simulink model "torque_controller_subsystem_completed_V2_R2019"  (R2019a)
settings: Solver=VariableStepAuto  StartTime=0.0  StopTime=5  RelTol=1e-3
model workspace (MAT data in the model file):
  DCBusVoltage = 24
  K_e = 221.0633
  L_d = 0.003482
  L_q = 0.00456
  Machine_Temperature = 25
  N = 9
  Peak_Current_String = 'Peak Current = 6.000000'
  PhaseAdvancesPerCycle = 36
  Phase_Advance_String = 'PhaseAdvance = 180.000000'
  PointsPerCycle = 36
  Rload = 1000000
  Rs = 0.624570538244
  Shaft_Speed = 27
  Sig = Simulink.Signal
  Sig.DataType = 'auto'
  Sig.Dimensions = -1
  Sig.DimensionsMode = 'auto'
  Sig.Complexity = 'auto'
  Sig.SampleTime = -1
  Sig.SamplingMode = 'auto'
  Sig1 = Simulink.Signal
  Sig1.DataType = 'auto'
  Sig1.Dimensions = -1
  Sig1.DimensionsMode = 'auto'
  Sig1.Complexity = 'auto'
  Sig1.SampleTime = -1
  Sig1.SamplingMode = 'auto'
  angleVec = [0 1.11111111111 2.22222222222 3.33333333333 4.44444444444 5.55555555556 6.66666666667 7.77777777778 8.88888888889 10 11.1111111111 12.2222222222 13.3333333333 14.4444444444 15.5555555556 16.6666666667 17.7777777778 18.8888888889 20 21.1111111111 22.2222222222 23.3333333333 24.4444444444 25.5555555556 26.6666666667 27.7777777778 28.8888888889 30 31.1111111111 32.2222222222 33.3333333333 34.4444444444 35.5555555556 36.6666666667 37.7777777778 38.8888888889 40]
  dq_inductance = 0.008366
  fluxAmat = [5.78758604472e-05 -0.00245230641441 -0.00496086974489 -0.00746825845512 -0.00997085180846 -0.0124701917234 -0.0149650380151 -0.0174527751443 -0.0199339133996 -0.0224017046643 -0.0248570910938 -0.0273006981398 ... (16428 elements, 12x37x37)]
  fluxD = 0.129208614948
  fluxDmat = [0.129332720835 0.129331856309 0.129330386347 0.129326055027 0.129320008491 0.129311398581 0.12929964601 0.129284600324 0.129267743431 0.129250546721 0.129230887735 0.129208614948 ... (16428 elements, 12x37x37)]
  fluxQ = -0.0273006981398
  fluxQmat = [5.78758604472e-05 -0.00245230641441 -0.00496086974489 -0.00746825845512 -0.00997085180846 -0.0124701917234 -0.0149650380151 -0.0174527751443 -0.0199339133996 -0.0224017046643 -0.0248570910938 -0.0273006981398 ... (16428 elements, 12x37x37)]
  fluxes = [-0.0273006981398; -0.0982475938625; 0.125548292002]
  funcresult = 0
  gammaVec = [-180 -170 -160 -150 -140 -130 -120 -110 -100 -90 -80 -70 -60 -50 -40 -30 -20 -10 0 10 20 30 40 50 60 70 80 90 100 110 120 130 140 150 160 170 180]
  i = 12
  invP = [-2.44929359829e-16  1; -0.866025403784  -0.5; 0.866025403784  -0.5]
  j = 37
  m = 37
  magVec = [0 0.545454545455 1.09090909091 1.63636363636 2.18181818182 2.72727272727 3.27272727273 3.81818181818 4.36363636364 4.90909090909 5.45454545455 6]
  nGamma = 37
  nMag = 12
  nX = 37
  poleNumber = 18
  pole_pairs = 9
  res1 = 0
  res2 = 0
  res3 = 0
  resistance_per_phase = 0.6246
  torque = -10.6713070894
  torqueMat = [-0.000127780443833 -0.972425785337 -1.94471415001 -2.91686171491 -3.8887574387 -4.86000619896 -5.83073162472 -6.80075888771 -7.77012767412 -8.7384579087 -9.70556312381 -10.6713070894 ... (16428 elements, 12x37x37)]
  torque_constant = 1.7505
  x1 = 360
  x2 = 360
  x3 = 360
  xe = 6.28318530718
  xlabel_string = 'Rotor angle (electrical °)'
  ylabel_string = 'Phase advance (°)'
libraries: fl_lib x12, nesl_utility x12, ee_lib x8, eeTransforms x3, simulink x2, powerlib_meascontrol x1
(part 1 of 2)
settings Model: OrderedModelArguments=off  Creator=mahdi  LastModifiedBy=mahdi
settings SolverCC: ZeroCrossAlgorithm=Adaptive

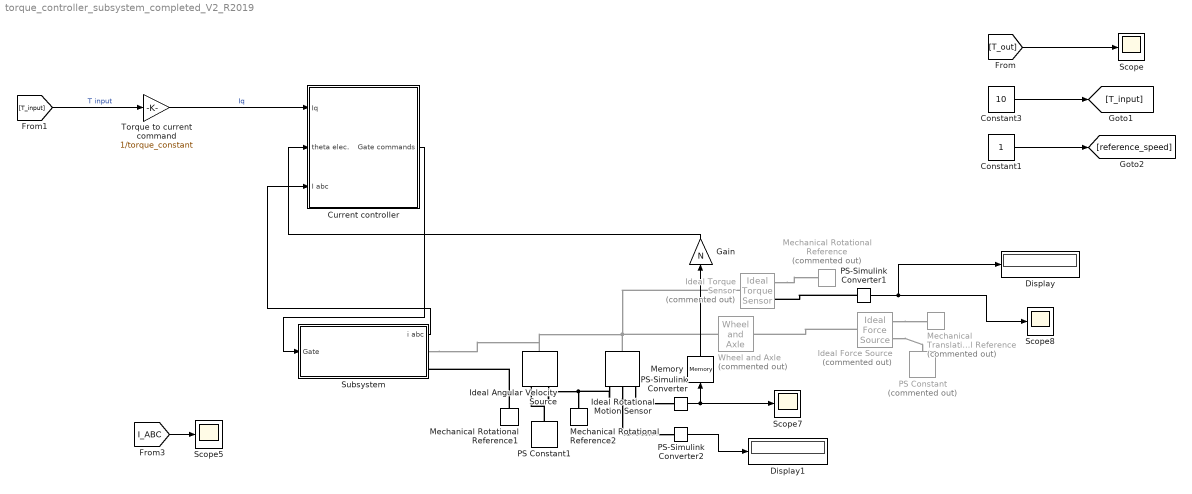
== system torque_controller_subsystem_completed_V2_R2019 ==
  Constant1 : Constant
  Constant3 : Constant  Value=10
  Current controller : Subsystem
  Display : Display
  Display1 : Display
  Gain : Gain  Gain=N
  Ideal Angular Velocity Source : fl_lib/Mechanical/Mechanical Sources/Ideal Angular Velocity Source
  Ideal Force Source : fl_lib/Mechanical/Mechanical Sources/Ideal Force Source  Commented=on
  Ideal Rotational Motion Sensor : fl_lib/Mechanical/Mechanical Sensors/Ideal Rotational Motion Sensor  wrap_angle=simscape.enum.onoff.off  offset=0 deg
      settings: SourceProductBaseCode=MT,SS
  Ideal Torque Sensor : fl_lib/Mechanical/Mechanical Sensors/Ideal Torque Sensor  Commented=on
  Mechanical Rotational Reference : fl_lib/Mechanical/Rotational Elements/Mechanical Rotational Reference  Commented=on
  Mechanical Rotational Reference1 : fl_lib/Mechanical/Rotational Elements/Mechanical Rotational Reference
      settings: SourceProductBaseCode=MT,SS
  Mechanical Rotational Reference2 : fl_lib/Mechanical/Rotational Elements/Mechanical Rotational Reference
      settings: SourceProductBaseCode=MT,SS
  Mechanical Translational Reference : fl_lib/Mechanical/Translational Elements/Mechanical Translational Reference  Commented=on
  Memory : Memory
  PS Constant : fl_lib/Physical Signals/Sources/PS Constant  Commented=on  constant=0
  PS Constant1 : fl_lib/Physical Signals/Sources/PS Constant  constant=1
  PS-Simulink Converter : nesl_utility/PS-Simulink Converter  PhysicalDomain=network_engine_domain  SubClassName=ps_output  LeftPortType=input  RightPortType=output  PseudoPeriodic=off  Frequencies=[]  Unit=inherit  AffineConversion=off
  PS-Simulink Converter1 : nesl_utility/PS-Simulink Converter  PhysicalDomain=network_engine_domain  SubClassName=ps_output  LeftPortType=input  RightPortType=output  PseudoPeriodic=off  Frequencies=[]  Unit=inherit  AffineConversion=off
  PS-Simulink Converter2 : nesl_utility/PS-Simulink Converter  PhysicalDomain=network_engine_domain  SubClassName=ps_output  LeftPortType=input  RightPortType=output  PseudoPeriodic=off  Frequencies=[]  Unit=inherit  AffineConversion=off
  Scope{,5,7..8} (4 alike) : Scope
  Subsystem : Subsystem
  Torque to current command : Gain  Gain=1/torque_constant
  Wheel and Axle : fl_lib/Mechanical/Mechanisms/Wheel and Axle  Commented=on  R=0.05 m  or=1  t_specify=off  t_priority=None  t=0 N*m  t_nominal_specify=off  t_nominal_unit=N*m  t_nominal_value=1  f_specify=off  f_priority=None  f=0 N  f_nominal_specify=off  f_nominal_unit=N  f_nominal_value=1
  wires:
  [T_input] -> Torque to current command/1  "T input"
  [T_out] -> Scope/1
  Constant3/1 -> [T_input]
  Constant1/1 -> [reference_speed]
  PS-Simulink Converter/1 -> Scope7/1, Memory/1
  PS-Simulink Converter1/1 -> Display/1, Scope8/1
  Memory/1 -> Gain/1
  PS-Simulink Converter2/1 -> Display1/1
  Torque to current command/1 -> Current controller/1(Iq)  "Iq"
  Gain/1 -> Current controller/2(theta elec.)
  Current controller/1(Gate commands) -> Subsystem/1(Gate)
  Subsystem/1(i abc) -> Current controller/3(I abc)
  [I_ABC] -> Scope5/1
  connections:
  Ideal Rotational Motion Sensor/RConn3 -- PS-Simulink Converter/LConn1
  Ideal Rotational Motion Sensor/RConn1 -- Ideal Angular Velocity Source/RConn2 -- Mechanical Rotational Reference2/LConn1
  Ideal Force Source/LConn1 -- Wheel and Axle/RConn1
  Ideal Force Source/RConn2 -- Mechanical Translational Reference/LConn1
  Ideal Force Source/RConn1 -- PS Constant/RConn1
  PS-Simulink Converter1/LConn1 -- Ideal Torque Sensor/RConn2
  Ideal Torque Sensor/LConn1 -- Subsystem/RConn1 -- Ideal Angular Velocity Source/LConn1 -- Wheel and Axle/LConn1 -- Ideal Rotational Motion Sensor/LConn1
  Ideal Torque Sensor/RConn1 -- Mechanical Rotational Reference/LConn1
  PS Constant1/RConn1 -- Ideal Angular Velocity Source/RConn1
  Ideal Rotational Motion Sensor/RConn2 -- PS-Simulink Converter2/LConn1
  Mechanical Rotational Reference1/LConn1 -- Subsystem/RConn2
